simulink model "doxeia"  (R2020a)
settings: Solver=VariableStepAuto  StartTime=0.0  StopTime=500  RelTol=1e-3
settings Model: Creator=bill2  LastModifiedBy=bill2
settings DataIOCC: Refine=10

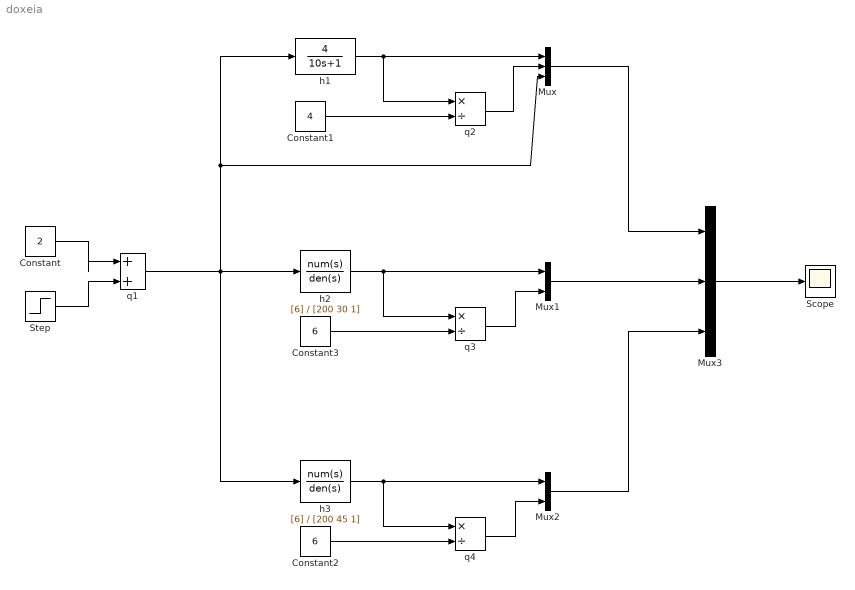
== system doxeia ==
  Constant : Constant  Value=2
  Constant1 : Constant  Value=4
  Constant2 : Constant  Value=6
  Constant3 : Constant  Value=6
  Mux : Mux  Inputs=3
  Mux1 : Mux  Inputs=2
  Mux2 : Mux  Inputs=2
  Mux3 : Mux  Inputs=3
  Scope : Scope
  Step : Step  Time=50  After=8  SampleTime=0
  h1 : TransferFcn  Numerator=[4]  Denominator=[10 1]
  h2 : TransferFcn  Numerator=[6]  Denominator=[200 30 1]
  h3 : TransferFcn  Numerator=[6]  Denominator=[200 45 1]
  q1 : Sum  Inputs=|++
  q2 : Product  Inputs=*/
  q3 : Product  Inputs=*/
  q4 : Product  Inputs=*/
  wires:
  Step/1 -> q1/2
  Constant/1 -> q1/1
  Constant1/1 -> q2/2
  h1/1 -> Mux/1, q2/1
  q1/1 -> h1/1, Mux/3, h3/1, h2/1
  Constant3/1 -> q3/2
  h2/1 -> Mux1/1, q3/1
  h3/1 -> q4/1, Mux2/1
  Constant2/1 -> q4/2
  Mux1/1 -> Mux3/2
  Mux/1 -> Mux3/1
  Mux3/1 -> Scope/1
  Mux2/1 -> Mux3/3
  q2/1 -> Mux/2
  q3/1 -> Mux1/2
  q4/1 -> Mux2/2
